simulink model "ActuatorSim"  (R2025b)
settings: Solver=FixedStepAuto  StartTime=0.0  StopTime=10.0  FixedStep=1/2000  RelTol=1e-3
values from neighbouring files (symbols this model uses):
  Cv = 16.5    [ActuatorModel.m]
  Km = 11    [ActuatorModel.m]
  m = m_a + 1/3 * m_p    (= 0.345333333333)    [ActuatorModel.m]
settings Model: Creator=thoma  LastModifiedBy=thoma

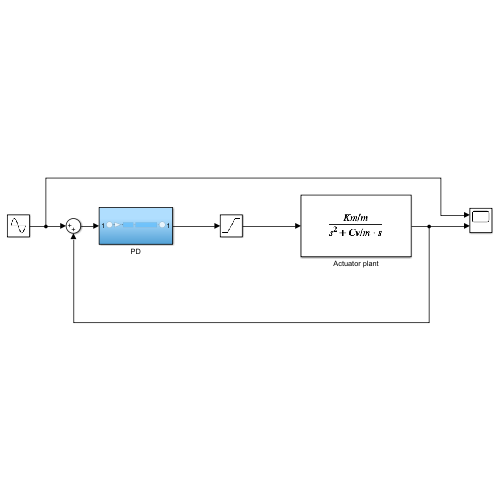
[thumbnail: Simulink's stored preview of the top-level diagram]
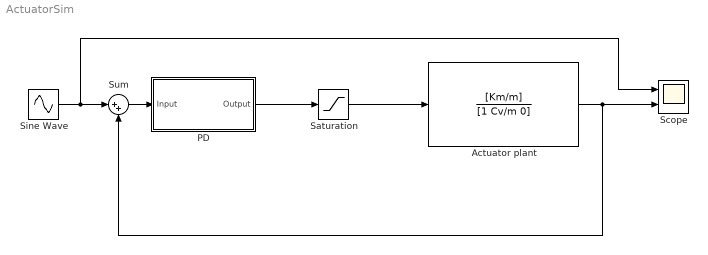
== system ActuatorSim ==
  Actuator plant : TransferFcn  Numerator=[Km/m]  Denominator=[1 Cv/m 0]
  PD : Subsystem
  Saturation : Saturate  UpperLimit=3  LowerLimit=-3
  Scope : Scope  NumInputPorts=2
      settings: ActiveDisplayYMinimum=-0.012462367849891492  ActiveDisplayYMaximum=0.019043618287474626
  Sine Wave : Sin  Amplitude=0.01  SampleTime=0
  Sum : Sum  Inputs=|++
  wires:
  PD/1(Output) -> Saturation/1
  Actuator plant/1 -> Sum/2, Scope/2
  Sine Wave/1 -> Scope/1, Sum/1
  Sum/1 -> PD/1(Input)
  Saturation/1 -> Actuator plant/1

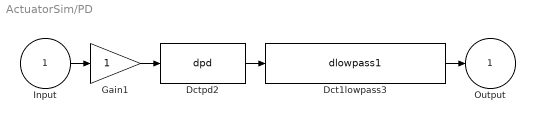
== system ActuatorSim/PD ==
  Input : Inport
  Dct1lowpass3 : S-Function  FunctionName=dlowpass1  Parameters=f_den, 0.001  SFunctionDeploymentMode=off  EnableBusSupport=off  mask(dctools){f_den=200}
      mask prompts: f_den "Pole [Hz]"
      mask help: This block implements a discrete time 1st order lowpass filter.
      mask Display: disp('DCT 1st order lowpass')
  Dctpd2 : S-Function  FunctionName=dpd  Parameters=kp, kv, 0.001  SFunctionDeploymentMode=off  EnableBusSupport=off  mask(dctools){kp=0.01, kv=10}
      mask help: This block implements a discrete time pd filter.
      mask Display: disp('DCT pd')
  Gain1 : Gain
  Output : Outport
  wires:
  Input/1 -> Gain1/1
  Gain1/1 -> Dctpd2/1
  Dctpd2/1 -> Dct1lowpass3/1
  Dct1lowpass3/1 -> Output/1
